simulink model "process_noise"  (R2023b)
settings: Solver=FixedStepAuto  StartTime=0.0  StopTime=0.2  FixedStep=0.2  RelTol=1e-3
values from neighbouring files (symbols this model uses):
  Phi = simulation.Phi(:,:,2)    [test_ProcessNoise.m]
  Propagation = data{2}    [test_ProcessNoise.m]
  R_bi = quat2rotm(q_m([4,1:3])')    [test_ProcessNoise.m]
undefined symbols (not defined in the file or in its folder): P_acc
libraries: nav_lib x1
settings Model: Creator=brent  LastModifiedBy=brent

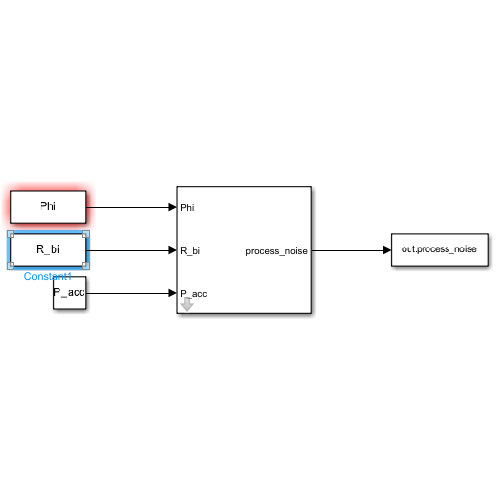
[thumbnail: Simulink's stored preview of the top-level diagram]
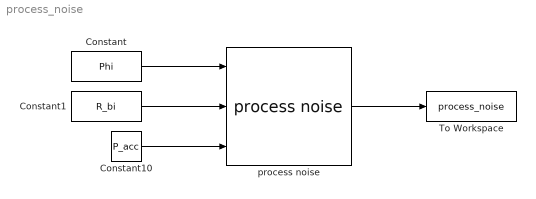
== system process_noise ==
  Constant : Constant  Value=Phi
  Constant1 : Constant  Value=R_bi
  Constant10 : Constant  Value=P_acc
  To Workspace : ToWorkspace  VariableName=process_noise  SampleTime=-1
  process noise : nav_lib/process noise  Q=Q.value  R_sb=R_sensor2body.value  dt=1/Propagation.lf.value
      settings: SourceProductName=Navigation library
  wires:
  process noise/1 -> To Workspace/1
  Constant1/1 -> process noise/2
  Constant10/1 -> process noise/3
  Constant/1 -> process noise/1
